simulink model "c_pvcm_2dof_ax1"  (R2024b)
settings: Solver=VariableStepAuto  StartTime=0.0  StopTime=10.0  RelTol=1e-3
values from neighbouring files (symbols this model uses):
  Ct = 1.0e4    (= 10000)    [simulate_root_locus.m]
  Dr = 0    [simulate_root_locus.m]
  FBtype = -1    [simulate_root_locus.m]
  Jr = 2.22e-3    (= 0.00222)    [simulate_root_locus.m]
  Kpp = Wvc/10    (= 40)    [simulate_root_locus.m]
  Kt = 1.1e8    (= 110000000)    [simulate_root_locus.m]
  KT = 1    [simulate_root_locus.m]
  Kvi = Wvc/5    (= 80)    [simulate_root_locus.m]
  Kvp = Ja*Wvc/KT    (= 10.88)    [simulate_root_locus.m]
  Mt = 500    [simulate_root_locus.m]
  pfb_on = 1    [simulate_root_locus.m]
  R = 3.2e-3    (= 0.0032)    [simulate_root_locus.m]
  vfb_on = 1    [simulate_root_locus.m]
settings Model: Creator=shohei  LastModifiedBy=shohei

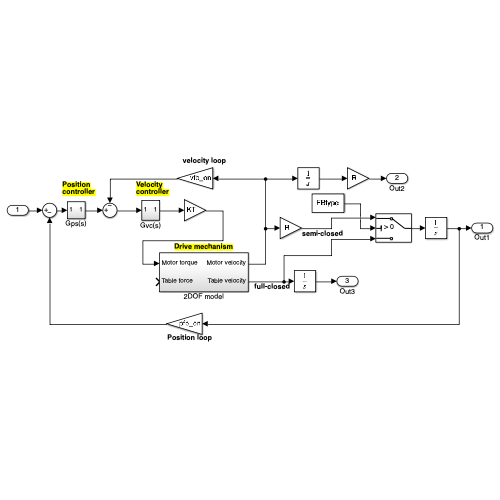
[thumbnail: Simulink's stored preview of the top-level diagram]
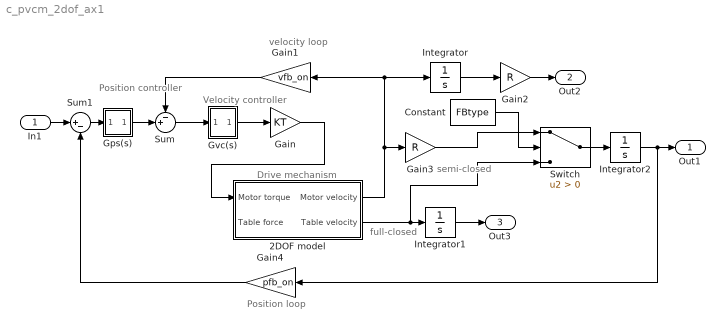
== system c_pvcm_2dof_ax1 ==
  note: Velocity
      | controller
  note: Position
      | controller
  note: velocity loop
  note: Position loop
  note: full-closed
  note: semi-closed
  note: Drive mechanism
  In1 : Inport
  2DOF model : Subsystem
  Constant : Constant  Value=FBtype
  Gain : Gain  Gain=KT
  Gain1 : Gain  Gain=vfb_on
  Gain2 : Gain  Gain=R
  Gain3 : Gain  Gain=R
  Gain4 : Gain  Gain=pfb_on
  Gps(s) : Subsystem
  Gvc(s) : Subsystem
  Integrator : Integrator
  Integrator1 : Integrator
  Integrator2 : Integrator
  Sum : Sum  Inputs=-+|
  Sum1 : Sum  Inputs=|+-
  Switch : Switch  Criteria=u2 > Threshold  SaturateOnIntegerOverflow=off  InputSameDT=off
  Out1 : Outport
  Out2 : Outport  Port=2
  Out3 : Outport  Port=3
  wires:
  Gvc(s)/1(Out1) -> Gain/1
  Gain/1 -> 2DOF model/1(Motor torque)
  Sum/1 -> Gvc(s)/1(In1)
  Gps(s)/1(Out1) -> Sum/2
  Gain1/1 -> Sum/1
  Integrator/1 -> Gain2/1
  2DOF model/1(Motor velocity) -> Integrator/1, Gain1/1, Gain3/1
  2DOF model/2(Table velocity) -> Switch/3, Integrator1/1
  Gain2/1 -> Out2/1
  Integrator1/1 -> Out3/1
  In1/1 -> Sum1/1
  Sum1/1 -> Gps(s)/1(In1)
  Gain4/1 -> Sum1/2
  Constant/1 -> Switch/2
  Gain3/1 -> Switch/1
  Switch/1 -> Integrator2/1
  Integrator2/1 -> Gain4/1, Out1/1

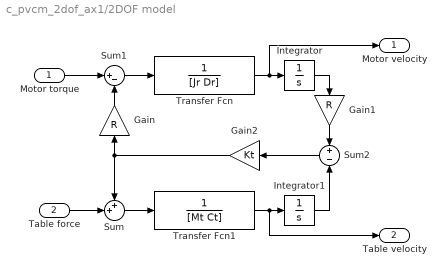
== system c_pvcm_2dof_ax1/2DOF model ==
  Motor torque : Inport
  Table force : Inport  Port=2
  Gain : Gain  Gain=R
  Gain1 : Gain  Gain=R
  Gain2 : Gain  Gain=Kt
  Integrator : Integrator
  Integrator1 : Integrator
  Sum : Sum  Inputs=++|
  Sum1 : Sum  Inputs=|+-
  Sum2 : Sum  Inputs=+|-
  Transfer Fcn : TransferFcn  Denominator=[Jr Dr]
  Transfer Fcn1 : TransferFcn  Denominator=[Mt Ct]
  Motor velocity : Outport
  Table velocity : Outport  Port=2
  wires:
  Integrator/1 -> Gain1/1
  Gain/1 -> Sum1/2
  Gain1/1 -> Sum2/1
  Sum/1 -> Transfer Fcn1/1
  Sum2/1 -> Gain2/1
  Integrator1/1 -> Sum2/2
  Transfer Fcn1/1 -> Table velocity/1, Integrator1/1
  Table force/1 -> Sum/2
  Transfer Fcn/1 -> Motor velocity/1, Integrator/1
  Motor torque/1 -> Sum1/1
  Sum1/1 -> Transfer Fcn/1
  Gain2/1 -> Sum/1, Gain/1

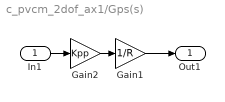
== system c_pvcm_2dof_ax1/Gps(s) ==
  In1 : Inport
  Gain1 : Gain  Gain=1/R
  Gain2 : Gain  Gain=Kpp
  Out1 : Outport
  wires:
  Gain2/1 -> Gain1/1
  In1/1 -> Gain2/1
  Gain1/1 -> Out1/1

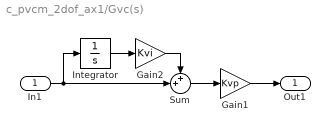
== system c_pvcm_2dof_ax1/Gvc(s) ==
  In1 : Inport
  Gain1 : Gain  Gain=Kvp
  Gain2 : Gain  Gain=Kvi
  Integrator : Integrator
  Sum : Sum  Inputs=++|
  Out1 : Outport
  wires:
  Integrator/1 -> Gain2/1
  In1/1 -> Integrator/1, Sum/2
  Sum/1 -> Gain1/1
  Gain1/1 -> Out1/1
  Gain2/1 -> Sum/1
